simulink model "Dynamics_RotationalEoM_TH"  (Simulink 7.8)
settings: Solver=ode45  StartTime=0.0  StopTime=10  RelTol=1e-3
libraries: AeroSim x1
settings Model: Creator=Ryan  LastModifiedBy=Ryan

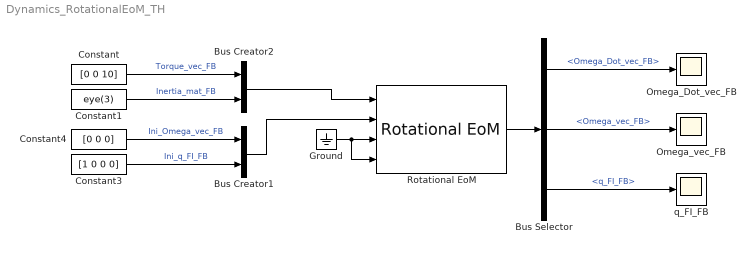
== system Dynamics_RotationalEoM_TH ==
  Bus Creator1 : BusCreator  Inputs=2
  Bus Creator2 : BusCreator  Inputs=2
  Bus Selector : BusSelector  OutputSignals=Omega_Dot_vec_FB,Omega_vec_FB,q_FI_FB
  Constant : Constant  Value=[0 0 10]
  Constant1 : Constant  Value=eye(3)
  Constant3 : Constant  Value=[1 0 0 0]
  Constant4 : Constant  Value=[0 0 0]
  Ground : Ground
  Omega_Dot_vec_FB : Scope
  Omega_vec_FB : Scope
  Rotational EoM : AeroSim/Dynamics/Rotational EoM
  q_FI_FB : Scope
      settings: SaveName=ScopeData2
  wires:
  Ground/1 -> Rotational EoM/4, Rotational EoM/3
  Constant/1 -> Bus Creator2/1  "Torque_vec_FB"
  Bus Creator2/1 -> Rotational EoM/1
  Bus Creator1/1 -> Rotational EoM/2
  Rotational EoM/1 -> Bus Selector/1
  Bus Selector/1 -> Omega_Dot_vec_FB/1  "<Omega_Dot_vec_FB>"
  Bus Selector/2 -> Omega_vec_FB/1  "<Omega_vec_FB>"
  Bus Selector/3 -> q_FI_FB/1  "<q_FI_FB>"
  Constant4/1 -> Bus Creator1/1  "Ini_Omega_vec_FB"
  Constant3/1 -> Bus Creator1/2  "Ini_q_FI_FB"
  Constant1/1 -> Bus Creator2/2  "Inertia_mat_FB"
